simulink model "pkg_ut"  (Simulink 8.1)
settings: Solver=FixedStepDiscrete  StartTime=0.0  StopTime=10.0  FixedStep=0.005  RelTol=1e-3
libraries: siltestlib x4, pkg x1
settings Model: Creator=xsellart  LastModifiedBy=AT015555
settings DataIOCC: SignalLoggingSaveFormat=Dataset
settings OptimizationCC: ExpressionDepthLimit=128
settings DebuggingCC: FcnCallInpInsideContextMsg=EnableAllAsError
settings GRTTargetCC: CombineOutputUpdateFcns=on  GRTInterface=off

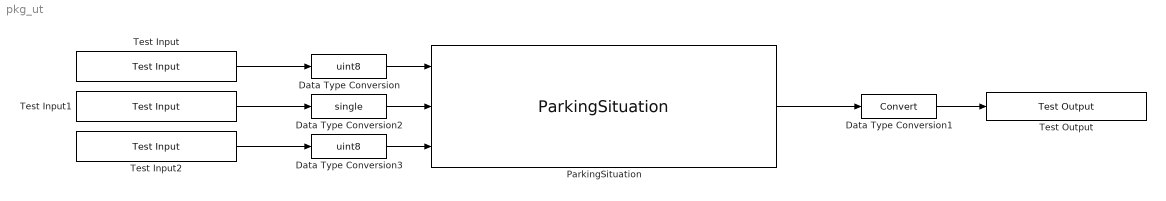
== system pkg_ut ==
  Data Type Conversion : DataTypeConversion  OutDataTypeStr=uint8
  Data Type Conversion1 : DataTypeConversion
  Data Type Conversion2 : DataTypeConversion  OutDataTypeStr=single
  Data Type Conversion3 : DataTypeConversion  OutDataTypeStr=uint8
  ParkingSituation : pkg/ParkingSituation
  Test Input : siltestlib/Test Input  varname=VDYN_GearPosition_enum  sampletime=0.005
  Test Input1 : siltestlib/Test Input  varname=VDINR_SteerAngle_deg  sampletime=0.005
  Test Input2 : siltestlib/Test Input  varname=VDINR_ParkBrakeBindSta_enum  sampletime=0.005
  Test Output : siltestlib/Test Output  varname=VIFO_ParkingSituation_flg  sampletime=-1
  wires:
  ParkingSituation/1 -> Data Type Conversion1/1
  Data Type Conversion1/1 -> Test Output/1
  Test Input/1 -> Data Type Conversion/1
  Data Type Conversion/1 -> ParkingSituation/1
  Test Input1/1 -> Data Type Conversion2/1
  Data Type Conversion2/1 -> ParkingSituation/2
  Test Input2/1 -> Data Type Conversion3/1
  Data Type Conversion3/1 -> ParkingSituation/3
